simulink model "sistema_sml"  (R2021a)
settings: Solver=VariableStepAuto  StartTime=0.0  StopTime=30  RelTol=1e-3
values from neighbouring files (symbols this model uses):
  T = 0    [sistema.m]
  tau1 = 0.001    [sistema.m]
  tau2 = 0.007    [sistema.m]
  x0 = 10    [sistema.m]
settings Model: Creator=halor  LastModifiedBy=halor

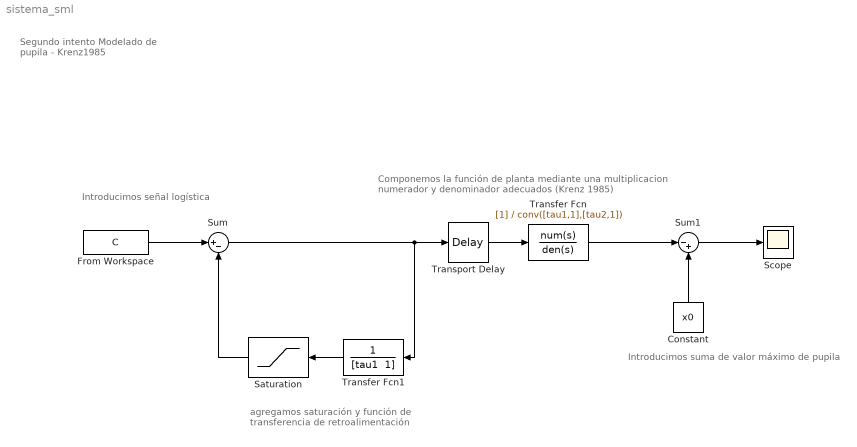
== system sistema_sml ==
  note: Introducimos suma de valor máximo de pupila
  note: Componemos la función de planta mediante una multiplicacion
      | numerador y denominador adecuados (Krenz 1985)
  note: agregamos saturación y función de
      | transferencia de retroalimentación
  note: Introducimos señal logística
  note: Segundo intento
      | Modelado de pupila - Krenz1985
  Constant : Constant  Value=x0
  From Workspace : FromWorkspace  VariableName=C
  Saturation : Saturate
  Scope : Scope
  Sum : Sum  Inputs=|+-
  Sum1 : Sum  Inputs=|-+
  Transfer Fcn : TransferFcn  Denominator=conv([tau1,1],[tau2,1])
  Transfer Fcn1 : TransferFcn  Denominator="[tau1  1]"
  Transport Delay : TransportDelay  DelayTime=T
  wires:
  Transfer Fcn/1 -> Sum1/1
  Sum/1 -> Transport Delay/1, Transfer Fcn1/1
  Transfer Fcn1/1 -> Saturation/1
  Saturation/1 -> Sum/2
  From Workspace/1 -> Sum/1
  Constant/1 -> Sum1/2
  Sum1/1 -> Scope/1
  Transport Delay/1 -> Transfer Fcn/1
